simulink model "try1"  (R2024a)
settings: Solver=FixedStepDiscrete  StartTime=0.0  StopTime=10.0  FixedStep=0.1  RelTol=1e-3
settings Model: Creator=DELL  LastModifiedBy=DELL

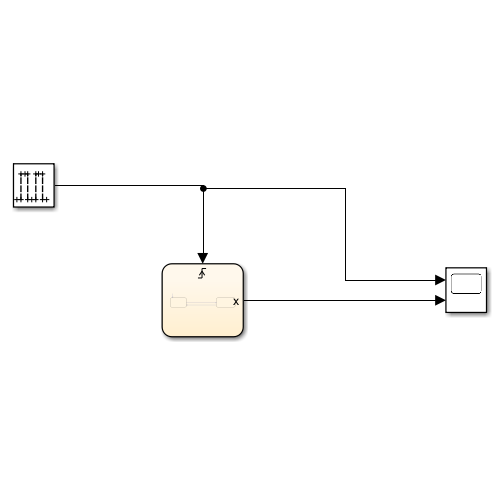
[thumbnail: Simulink's stored preview of the top-level diagram]
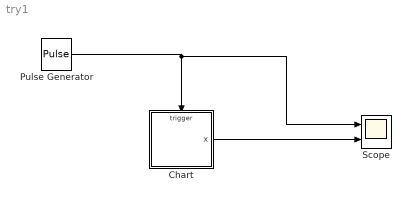
== system try1 ==
  Chart : Stateflow chart  TreatAsAtomicUnit=on
  Pulse Generator : DiscretePulseGenerator  Period=5  PulseWidth=2  SampleTime=0.1
  Scope : Scope  NumInputPorts=2
  wires:
  Chart/1(x) -> Scope/2
  Pulse Generator/1 -> Scope/1, Chart/Trigger

== stateflow chart try1/Chart ==
  settings: executeAtInitialization=1
  state one
    en:
    x=6;
  state two
    en:
    x=3;
  (default) -> one
  one -> two : event
  two -> one : event
  data: x output
  events: event input RISING_EDGE_EVENT
